simulink model "lab753_usrp_qpsk"  (R2018b)
settings: Solver=VariableStepAuto  StartTime=0.0  StopTime=inf  RelTol=1e-3
libraries: dspmlti4 x3, dspfdesign x3, commrandsrc3 x1, commdigbbndpm3 x1, commfilt2 x1, commsdrhw_v2 x1
settings Model: Creator=Григорий Фокин  LastModifiedBy=Григорий Фокин

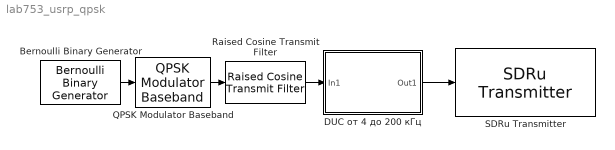
== system lab753_usrp_qpsk ==
  Bernoulli Binary Generator : commrandsrc3/Bernoulli Binary Generator  ProbabilityOfZero=0.5  SeedSource=Parameter  Seed=61  SampleTime=1/2e3  SamplesPerFrame=2  OutputDataType=boolean  SimulateUsing=Interpreted execution
  "DUC от 4 до 200 кГц " : Subsystem
  QPSK Modulator Baseband : commdigbbndpm3/QPSK Modulator Baseband  InType=Bit  Enc=Gray  Ph=pi/4  outDtype=double  outWordLen=16  outUDDataType=sfix(16)  outFracLenMode=Best precision  outFracLen=15  outDataTypeStr=double  outLastDataTypeStr=double
  Raised Cosine Transmit Filter : commfilt2/Raised Cosine Transmit Filter  filtType=Square root  R=0.5  filtSpan=12  N=4  filterGain=1  InputProcessing=Columns as channels (frame based)  RateOptions=Allow multirate processing  framing=Mute  checkCoeff=off  variableName=rcTxFilt  checkGain=Normalized  sampMode=Mute  saveAsFlag=0  currentFiltSpan=12  D=(12)/2  launchFVT=on  roundingMode=Floor  overflowMode=off  coeffDataTypeStr=Inherit: Same word length as input  coeffMin=[]  coeffMax=[]  coeffLastDataTypeStr=Inherit: Same word length as input  outputDataTypeStr=Inherit: Same as accumulator  outputMin=[]  outputMax=[]  outputLastDataTypeStr=Inherit: Same as accumulator
  SDRu Transmitter : commsdrhw_v2/SDRu Transmitter  rxtx=tx  initializeIPAddress=0  devMap=0  USRP2_IP=192.168.10.2  USRP_IP_X300=192.168.10.2  USRP_IP_X310=192.168.10.2  USRP_serialNumB200=No devices found  USRP_serialNumB210=F4E642  platform=B210  prevPlatform=B210  lastIPAddressPopup=192.168.10.2  USRP_ID=F4E642  LastIPAddress=192.168.10.2  ChannelMapping=1  centerFrequencySrc=Dialog  centerFrequency=1200e6  loOffsetSrc=Dialog  loOffset=250e3  gainSrc=Dialog  gain=70  PPSSource=Internal  clockSource=Internal  masterClkRateParam=6000000  masterClkRateB200=32e6  masterClkRateB210=6e6  masterClkRateX300=120e6  masterClkRateX310=120e6  decimInterpSrc=Dialog  decimInterp=30  USRP2_IP_NUM=[70 52 69 54 52 50]  frameLength=362  TransportDataType=int16  outputDatatype=Same as transport data type  overrunUnderrunPort=off  sampleTime=1  dboardInfo=|  HOST_DATA_PORT=30000  HOST_CONTROL_PORT=30001  USRP2_DATA_PORT=32769  USRP2_CONTROL_PORT=32768  bufferMode=Continuous streaming  EnableBurstMode=off  NumFramesInBurst=100
      | dbid: 0
      |           dbName: 'no db found'
      |          freqMin: 0
      |          freqMax: 0
      |          gainMin: 0
      |          gainMax: 0
      |     gainStepSize: 0
      settings: SourceProductName=Communications System Toolbox Support Package for USRP(R) Radio  SourceProductBaseCode=USRP
  wires:
  Bernoulli Binary Generator/1 -> QPSK Modulator Baseband/1
  QPSK Modulator Baseband/1 -> Raised Cosine Transmit Filter/1
  Raised Cosine Transmit Filter/1 -> "DUC от 4 до 200 кГц "/1(In1)
  "DUC от 4 до 200 кГц "/1(Out1) -> SDRu Transmitter/1

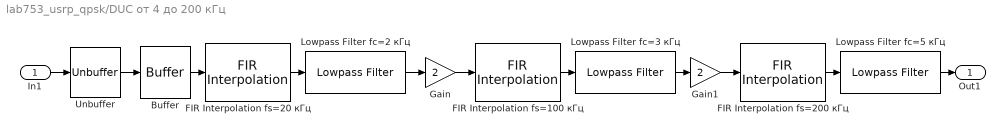
== system lab753_usrp_qpsk/DUC от 4 до 200 кГц  ==
  In1 : Inport
  Buffer : Buffer  N=1000  OutputFrames=off
  FIR Interpolation fs=100 кГц : dspmlti4/FIR Interpolation  FilterSource=Dialog parameters  h=firpm(75,[0 5e3 10e3 100e3/2]/(100e3/2), [1 1 0 0], [1 1], 20)  L=5  FilterObject=FINTERP  InputProcessing=Columns as channels (frame based)  framing=Allow multirate processing  outputBufInitCond=0  roundingMode=Floor  overflowMode=off  firstCoeffDataTypeStr=Inherit: Same word length as input  firstCoeffMin=[]  firstCoeffMax=[]  firstCoeffLastDataTypeStr=Inherit: Same word length as input  outputDataTypeStr=Inherit: Same as accumulator  outputMin=[]  outputMax=[]  outputLastDataTypeStr=Inherit: Same as accumulator
      settings: SourceProductName=DSP System Toolbox
  FIR Interpolation fs=20 кГц : dspmlti4/FIR Interpolation  FilterSource=Dialog parameters  h=firpm(75,[0 1.5e3 2e3 20e3/2]/(20e3/2), [1 1 0 0], [1 1], 20)  L=5  FilterObject=FINTERP  InputProcessing=Columns as channels (frame based)  framing=Allow multirate processing  outputBufInitCond=0  roundingMode=Floor  overflowMode=off  firstCoeffDataTypeStr=Inherit: Same word length as input  firstCoeffMin=[]  firstCoeffMax=[]  firstCoeffLastDataTypeStr=Inherit: Same word length as input  outputDataTypeStr=Inherit: Same as accumulator  outputMin=[]  outputMax=[]  outputLastDataTypeStr=Inherit: Same as accumulator
      settings: SourceProductName=DSP System Toolbox
  FIR Interpolation fs=200 кГц : dspmlti4/FIR Interpolation  FilterSource=Dialog parameters  h=firpm(75,[0 5e3 15e3 200e3/2]/(200e3/2), [1 1 0 0], [1 1], 20)  L=2  FilterObject=FINTERP  InputProcessing=Columns as channels (frame based)  framing=Allow multirate processing  outputBufInitCond=0  roundingMode=Floor  overflowMode=off  firstCoeffDataTypeStr=Inherit: Same word length as input  firstCoeffMin=[]  firstCoeffMax=[]  firstCoeffLastDataTypeStr=Inherit: Same word length as input  outputDataTypeStr=Inherit: Same as accumulator  outputMin=[]  outputMax=[]  outputLastDataTypeStr=Inherit: Same as accumulator
      settings: SourceProductName=DSP System Toolbox
  Gain : Gain  Gain=2
  Gain1 : Gain  Gain=2
  Lowpass Filter fc=2 кГц : dspfdesign/Lowpass Filter  FilterType=FIR  DesignForMinimumOrder=on  FilterOrder=50  PassbandFrequency=2e3  StopbandFrequency=3e3  PassbandRipple=0.1  StopbandAttenuation=80  InheritSampleRate=off  SampleRate=20e3  SimulateUsing=Interpreted execution  roundingMode=Floor  coeffsDataTypeStr=fixdt(1,16)
  Lowpass Filter fc=3 кГц : dspfdesign/Lowpass Filter  FilterType=FIR  DesignForMinimumOrder=on  FilterOrder=50  PassbandFrequency=3e3  StopbandFrequency=10e3  PassbandRipple=0.1  StopbandAttenuation=80  InheritSampleRate=off  SampleRate=100e3  SimulateUsing=Interpreted execution  roundingMode=Floor  coeffsDataTypeStr=fixdt(1,16)
  Lowpass Filter fc=5 кГц : dspfdesign/Lowpass Filter  FilterType=FIR  DesignForMinimumOrder=on  FilterOrder=50  PassbandFrequency=5e3  StopbandFrequency=15e3  PassbandRipple=0.1  StopbandAttenuation=80  InheritSampleRate=off  SampleRate=200e3  SimulateUsing=Interpreted execution  roundingMode=Floor  coeffsDataTypeStr=fixdt(1,16)
  Unbuffer : Unbuffer
  Out1 : Outport
  wires:
  Lowpass Filter fc=2 кГц/1 -> Gain/1
  FIR Interpolation fs=100 кГц/1 -> Lowpass Filter fc=3 кГц/1
  FIR Interpolation fs=20 кГц/1 -> Lowpass Filter fc=2 кГц/1
  Lowpass Filter fc=5 кГц/1 -> Out1/1
  Lowpass Filter fc=3 кГц/1 -> Gain1/1
  FIR Interpolation fs=200 кГц/1 -> Lowpass Filter fc=5 кГц/1
  Buffer/1 -> FIR Interpolation fs=20 кГц/1
  In1/1 -> Unbuffer/1
  Unbuffer/1 -> Buffer/1
  Gain/1 -> FIR Interpolation fs=100 кГц/1
  Gain1/1 -> FIR Interpolation fs=200 кГц/1
